simulink model "dtc_svpwm"  (Simulink 7.0)
settings: Solver=ode23tb  StartTime=0.0  StopTime=0.1  RelTol=1e-3
libraries: powerlib x4
settings Model: Creator=Administrator  LastModifiedBy=Administrator
settings SolverCC: ZeroCrossControl=DisableAll

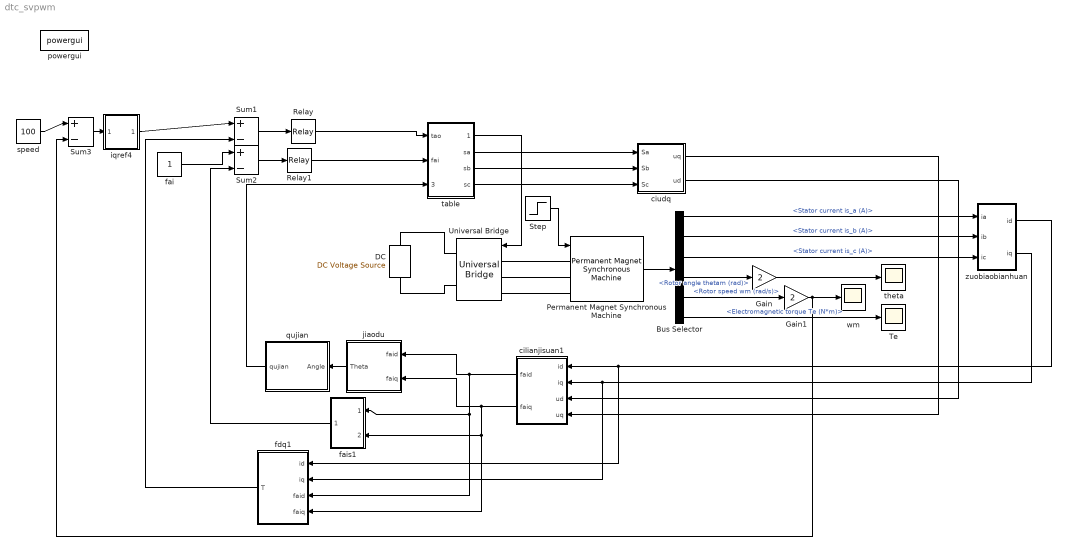
== system dtc_svpwm ==
  Bus Selector : BusSelector  OutputSignals=Stator current is_a (A),Stator current is_b (A),Stator current is_c (A),Rotor angle thetam (rad),Rotor speed wm (rad/s),Electromagnetic torque Te (N*m)
  "DC " : powerlib/Electrical Sources/DC Voltage Source  Orientation=up  DialogController=POWERSYS.PowerSysDialog  SystemSampleTime=-1  Amplitude=310  Measurements=None
  Gain : Gain  Gain=2  ParameterDataType=sfix(16)  ParameterScaling=2^0  OutDataType=sfix(16)  OutScaling=2^0
  Gain1 : Gain  Gain=2  ParameterDataType=sfix(16)  ParameterScaling=2^0  OutDataType=sfix(16)  OutScaling=2^0
  Permanent Magnet Synchronous Machine : powerlib/Machines/Permanent Magnet Synchronous Machine  DialogController=POWERSYS.PowerSysDialog  SystemSampleTime=-1  FluxDistribution=Sinusoidal  MechanicalLoad=Torque Tm  PresetModel=No  ShowDetailedParameters=on  Resistance=2.8750  Inductance=8.5e-3  dqInductances=[8.5e-3;8.5e-3]  Flux=0.3  Flat=120  Mechanical=[0.008 0 2]  PolePairs=2
  Relay : Relay  OnSwitchValue=0.001  OffSwitchValue=-0.001  OutDataType=sfix(16)  OutScaling=2^0
  Relay1 : Relay  OnSwitchValue=0.005  OffSwitchValue=-0.005  OutDataType=sfix(16)  OutScaling=2^0
  Step : Step  Time=0.04  Before=1  After=2  SampleTime=0
  Sum1 : Sum  Inputs=|+-  OutDataType=sfix(16)  OutScaling=2^0
  Sum2 : Sum  Inputs=|+-  OutDataType=sfix(16)  OutScaling=2^0
  Sum3 : Sum  Inputs=|+-  OutDataType=sfix(16)  OutScaling=2^0
  Te : Scope
      settings: YMin=-50  YMax=55
  Universal Bridge : powerlib/Power Electronics/Universal Bridge  Orientation=left  DialogController=POWERSYS.PowerSysDialog  SystemSampleTime=-1  Arms=3  SnubberResistance=1e5  SnubberCapacitance=inf  Device=IGBT / Diodes  Ron=1e-3  Lon=0  ForwardVoltages="[  0  0  ]"  ForwardVoltage=0  GTOparameters=[ 10e-6 , 20e-6 ]  IGBTparameters=[ 1e-6 , 2e-6 ]  Measurements=None  converterType=Rectifier
  cilianjisuan1 : Subsystem  Orientation=left
  ciudq : Subsystem
  fai : Constant  OutDataType=sfix(16)  OutScaling=2^0
  fais1 : Subsystem  Orientation=left
  fdq1 : Subsystem  Orientation=left
  iqref4 : Subsystem  mask(PI Controller){@1=0.02, @2=2, @3=[-3000, 3000]}
      mask prompts: @1 "Integral"; @2 "Proportional:"; @3 "Minimum and maximum outputs:"
      mask init:
      | I=@1;P=@2;sat=@3;min=sat(1);max=sat(2);
      mask Display: disp('PI')
  jiaodu : Subsystem  Orientation=left
  powergui : powerlib/powergui  SystemSampleTime=-1  SimulationMode=Continuous  SampleTime=50e-6  echomessages=off  RestoreLinks=warning  x0status=blocks  Frange=[0:2:500]  Ylog=off  Xlog=on  ShowGrid=off  save=off  variable=ZData  ZoomFFT=on  StartTime=0.0  cycles=1  DisplayStyle=1  fundamental=60  FreqAxis=off  MaxFrequency=1000  frequencyindice=0  frequencyindicesteady=1  RmsSteady=1  display=off  Ts=0  frequency=60  methode=off  HookPort=off  Interpol=off  SPID=off  FunctionMessages=off
  qujian : Subsystem  Orientation=left
  speed : Constant  Value=100  OutDataType=sfix(16)  OutScaling=2^0
  table : Subsystem
  theta : Scope
      settings: SaveName=ScopeData2
  wm : Scope
      settings: YMin=-100  YMax=110  SaveName=ScopeData3
  zuobiaobianhuan : Subsystem
      mask Type: bianhuan
  wires:
  table/1(Pulse) -> Universal Bridge/1
  Permanent Magnet Synchronous Machine/1 -> Bus Selector/1
  Bus Selector/4 -> Gain/1  "<Rotor angle thetam (rad)>"
  Gain/1 -> theta/1
  Bus Selector/6 -> Te/1  "<Electromagnetic torque Te (N*m)>"
  Gain1/1 -> wm/1, Sum3/2
  Step/1 -> Permanent Magnet Synchronous Machine/1
  Sum1/1 -> Relay/1
  Sum2/1 -> Relay1/1
  fais1/1(fais) -> Sum2/2
  fai/1 -> Sum2/1
  fdq1/1(T) -> Sum1/2
  jiaodu/1(Theta) -> qujian/1(Angle)
  cilianjisuan1/1(faid) -> jiaodu/1(faid), fdq1/3(faid), fais1/1(faid)
  cilianjisuan1/2(faiq) -> jiaodu/2(faiq), fdq1/4(faiq), fais1/2(faiq)
  table/3(sb) -> ciudq/2(Sb)
  speed/1 -> Sum3/1
  Bus Selector/5 -> Gain1/1  "<Rotor speed wm (rad/s)>"
  table/2(sa) -> ciudq/1(Sa)
  table/4(sc) -> ciudq/3(Sc)
  zuobiaobianhuan/1(id) -> fdq1/1(id), cilianjisuan1/1(id)
  zuobiaobianhuan/2(iq) -> fdq1/2(iq), cilianjisuan1/2(iq)
  Bus Selector/1 -> zuobiaobianhuan/1(ia)  "<Stator current is_a (A)>"
  Bus Selector/2 -> zuobiaobianhuan/2(ib)  "<Stator current is_b (A)>"
  Bus Selector/3 -> zuobiaobianhuan/3(ic)  "<Stator current is_c (A)>"
  Relay/1 -> table/1(tao)
  Relay1/1 -> table/2(fai)
  qujian/1(qujian) -> table/3(theta)
  Sum3/1 -> iqref4/1(In_1)
  iqref4/1(Out_1) -> Sum1/1
  ciudq/1(uq) -> cilianjisuan1/4(uq)
  ciudq/2(ud) -> cilianjisuan1/3(ud)
  connections:
  "DC "/RConn1 -- Universal Bridge/RConn1
  "DC "/LConn1 -- Universal Bridge/RConn2
  Universal Bridge/LConn1 -- Permanent Magnet Synchronous Machine/LConn1
  Universal Bridge/LConn2 -- Permanent Magnet Synchronous Machine/LConn2
  Universal Bridge/LConn3 -- Permanent Magnet Synchronous Machine/LConn3

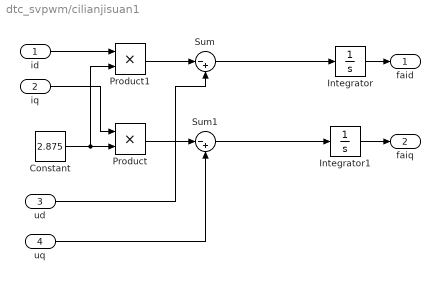
== system dtc_svpwm/cilianjisuan1 ==
  id : Inport  OutDataType=sfix(16)  OutScaling=2^0
  iq : Inport  Port=2  OutDataType=sfix(16)  OutScaling=2^0
  ud : Inport  Port=3  OutDataType=sfix(16)  OutScaling=2^0
  uq : Inport  Port=4  OutDataType=sfix(16)  OutScaling=2^0
  Constant : Constant  Value=2.875  OutDataType=sfix(16)  OutScaling=2^0
  Integrator : Integrator  InitialCondition=0.01
  Integrator1 : Integrator  InitialCondition=0.01
  Product : Product  OutDataType=sfix(16)  OutScaling=2^0  RndMeth=Zero
  Product1 : Product  OutDataType=sfix(16)  OutScaling=2^0  RndMeth=Zero
  Sum : Sum  Inputs=|-+  OutDataType=sfix(16)  OutScaling=2^0
  Sum1 : Sum  Inputs=|-+  OutDataType=sfix(16)  OutScaling=2^0
  faid : Outport  OutDataType=sfix(16)  OutScaling=2^0
  faiq : Outport  Port=2  OutDataType=sfix(16)  OutScaling=2^0
  wires:
  Integrator/1 -> faid/1
  Sum/1 -> Integrator/1
  Integrator1/1 -> faiq/1
  Sum1/1 -> Integrator1/1
  iq/1 -> Product/1
  Constant/1 -> Product/2, Product1/2
  id/1 -> Product1/1
  Product1/1 -> Sum/1
  Product/1 -> Sum1/1
  ud/1 -> Sum/2
  uq/1 -> Sum1/2

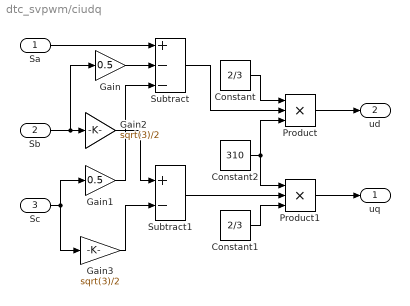
== system dtc_svpwm/ciudq ==
  Sa : Inport
  Sb : Inport  Port=2
  Sc : Inport  Port=3
  Constant : Constant  Value=2/3
  Constant1 : Constant  Value=2/3
  Constant2 : Constant  Value=310
  Gain : Gain  Gain=0.5
  Gain1 : Gain  Gain=0.5
  Gain2 : Gain  Gain=sqrt(3)/2
  Gain3 : Gain  Gain=sqrt(3)/2
  Product : Product  Inputs=3  RndMeth=Zero
  Product1 : Product  Inputs=3  RndMeth=Zero
  Subtract : Sum  Inputs=+--
  Subtract1 : Sum  Inputs=+-
  uq : Outport
  ud : Outport  Port=2
  wires:
  Sa/1 -> Subtract/1
  Gain/1 -> Subtract/2
  Sb/1 -> Gain2/1, Gain/1
  Sc/1 -> Gain3/1, Gain1/1
  Gain1/1 -> Subtract/3
  Gain2/1 -> Subtract1/1
  Gain3/1 -> Subtract1/2
  Subtract/1 -> Product/2
  Constant/1 -> Product/1
  Subtract1/1 -> Product1/2
  Constant1/1 -> Product1/3
  Constant2/1 -> Product1/1, Product/3
  Product/1 -> ud/1
  Product1/1 -> uq/1

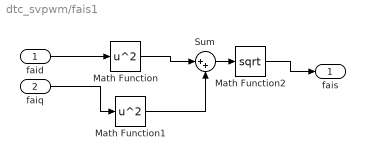
== system dtc_svpwm/fais1 ==
  faid : Inport  OutDataType=sfix(16)  OutScaling=2^0
  faiq : Inport  Port=2  OutDataType=sfix(16)  OutScaling=2^0
  Math Function : Math  Operator=square  OutDataType=sfix(16)  OutScaling=2^0  SaturateOnIntegerOverflow=on
  Math Function1 : Math  Operator=square  OutDataType=sfix(16)  OutScaling=2^0  SaturateOnIntegerOverflow=on
  Math Function2 : Math  Operator=sqrt  OutDataType=sfix(16)  OutScaling=2^0  SaturateOnIntegerOverflow=on
  Sum : Sum  Inputs=|++  OutDataType=sfix(16)  OutScaling=2^0
  fais : Outport  OutDataType=sfix(16)  OutScaling=2^0
  wires:
  faid/1 -> Math Function/1
  faiq/1 -> Math Function1/1
  Math Function2/1 -> fais/1
  Math Function/1 -> Sum/1
  Math Function1/1 -> Sum/2
  Sum/1 -> Math Function2/1

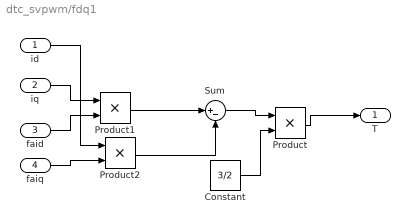
== system dtc_svpwm/fdq1 ==
  id : Inport  OutDataType=sfix(16)  OutScaling=2^0
  iq : Inport  Port=2  OutDataType=sfix(16)  OutScaling=2^0
  faid : Inport  Port=3  OutDataType=sfix(16)  OutScaling=2^0
  faiq : Inport  Port=4  OutDataType=sfix(16)  OutScaling=2^0
  Constant : Constant  Value=3/2  OutDataType=sfix(16)  OutScaling=2^0
  Product : Product  OutDataType=sfix(16)  OutScaling=2^0  RndMeth=Zero
  Product1 : Product  OutDataType=sfix(16)  OutScaling=2^0  RndMeth=Zero
  Product2 : Product  OutDataType=sfix(16)  OutScaling=2^0  RndMeth=Zero
  Sum : Sum  Inputs=|+-  OutDataType=sfix(16)  OutScaling=2^0
  T : Outport  OutDataType=sfix(16)  OutScaling=2^0
  wires:
  Sum/1 -> Product/1
  Constant/1 -> Product/2
  Product/1 -> T/1
  iq/1 -> Product1/1
  faid/1 -> Product1/2
  id/1 -> Product2/1
  faiq/1 -> Product2/2
  Product2/1 -> Sum/2
  Product1/1 -> Sum/1

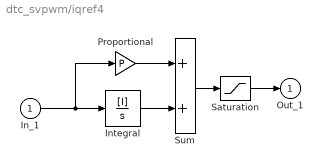
== system dtc_svpwm/iqref4 ==
  In_1 : Inport  OutDataType=sfix(16)  OutScaling=2^0
  Integral : TransferFcn  Numerator=[I]  Denominator=[1 0]
  Proportional : Gain  Gain=P  ParameterDataType=sfix(16)  ParameterScaling=2^0  OutDataType=sfix(16)  OutScaling=2^0  SaturateOnIntegerOverflow=on
  Saturation : Saturate  UpperLimit=max  LowerLimit=min
  Sum : Sum  OutDataType=sfix(16)  OutScaling=2^0  SaturateOnIntegerOverflow=on  InputSameDT=on
  Out_1 : Outport  OutDataType=sfix(16)  OutScaling=2^0  InitialOutput=0
  wires:
  Saturation/1 -> Out_1/1
  Sum/1 -> Saturation/1
  Proportional/1 -> Sum/1
  In_1/1 -> Proportional/1, Integral/1
  Integral/1 -> Sum/2

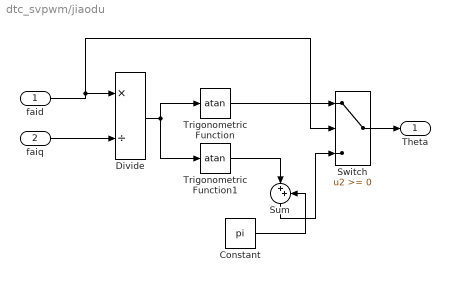
== system dtc_svpwm/jiaodu ==
  faid : Inport  OutDataType=sfix(16)  OutScaling=2^0
  faiq : Inport  Port=2  OutDataType=sfix(16)  OutScaling=2^0
  Constant : Constant  Value=pi  OutDataType=sfix(16)  OutScaling=2^0
  Divide : Product  Inputs=*/  OutDataType=sfix(16)  OutScaling=2^-10
  Sum : Sum  Orientation=down  Inputs=|++  OutDataType=sfix(16)  OutScaling=2^0
  Switch : Switch  OutDataType=sfix(16)  OutScaling=2^0
  Trigonometric Function : Trigonometry  Operator=atan
  Trigonometric Function1 : Trigonometry  Operator=atan
  Theta : Outport  OutDataType=sfix(16)  OutScaling=2^0
  wires:
  faid/1 -> Divide/1, Switch/2
  faiq/1 -> Divide/2
  Trigonometric Function/1 -> Switch/1
  Sum/1 -> Switch/3
  Constant/1 -> Sum/2
  Switch/1 -> Theta/1
  Divide/1 -> Trigonometric Function1/1, Trigonometric Function/1
  Trigonometric Function1/1 -> Sum/1

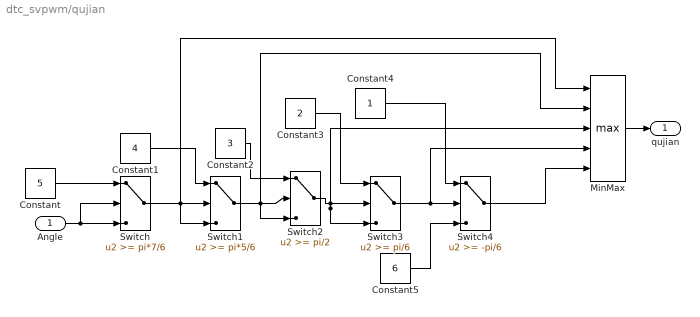
== system dtc_svpwm/qujian ==
  Angle : Inport  OutDataType=sfix(16)  OutScaling=2^0
  Constant : Constant  Value=5  OutDataType=sfix(16)  OutScaling=2^0
  Constant1 : Constant  Value=4  OutDataType=sfix(16)  OutScaling=2^0
  Constant2 : Constant  Value=3  OutDataType=sfix(16)  OutScaling=2^0
  Constant3 : Constant  Value=2  OutDataType=sfix(16)  OutScaling=2^0
  Constant4 : Constant  OutDataType=sfix(16)  OutScaling=2^0
  Constant5 : Constant  Value=6  OutDataType=sfix(16)  OutScaling=2^0
  MinMax : MinMax  Function=max  Inputs=5  OutDataType=sfix(16)  OutScaling=2^0
  Switch : Switch  Threshold=pi*7/6  OutDataType=sfix(16)  OutScaling=2^0
  Switch1 : Switch  Threshold=pi*5/6  OutDataType=sfix(16)  OutScaling=2^0
  Switch2 : Switch  Threshold=pi/2  OutDataType=sfix(16)  OutScaling=2^0
  Switch3 : Switch  Threshold=pi/6  OutDataType=sfix(16)  OutScaling=2^0
  Switch4 : Switch  Threshold=-pi/6  OutDataType=sfix(16)  OutScaling=2^0
  qujian : Outport  OutDataType=sfix(16)  OutScaling=2^0
  wires:
  Angle/1 -> Switch/3, Switch/2
  Constant/1 -> Switch/1
  Switch/1 -> Switch1/2, Switch1/3, MinMax/1
  Switch1/1 -> MinMax/2, Switch2/2, Switch2/3
  Constant1/1 -> Switch1/1
  Constant2/1 -> Switch2/1
  Constant3/1 -> Switch3/1
  Switch4/1 -> MinMax/5
  Constant4/1 -> Switch4/1
  MinMax/1 -> qujian/1
  Constant5/1 -> Switch4/3
  Switch2/1 -> Switch3/2, Switch3/3, MinMax/3
  Switch3/1 -> Switch4/2, MinMax/4

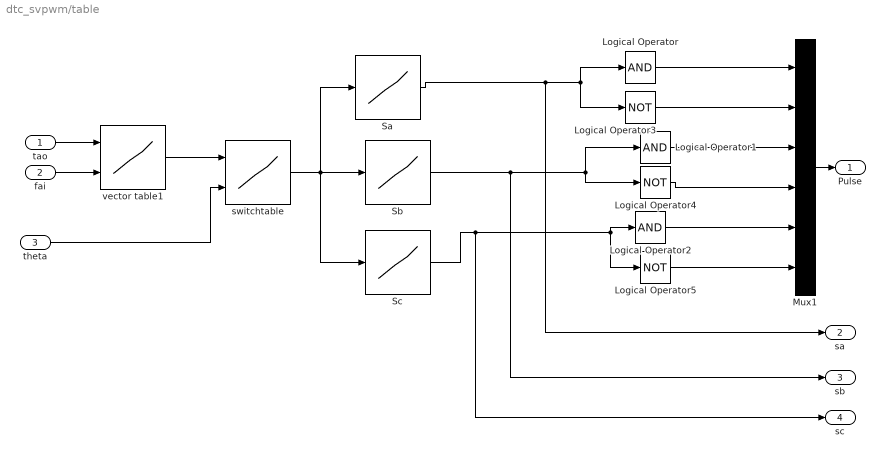
== system dtc_svpwm/table ==
  tao : Inport  OutDataType=sfix(16)  OutScaling=2^0
  fai : Inport  Port=2  OutDataType=sfix(16)  OutScaling=2^0
  theta : Inport  Port=3  OutDataType=sfix(16)  OutScaling=2^0
  Logical Operator : Logic  Inputs=1  AllPortsSameDT=off  OutDataTypeMode=boolean
  Logical Operator1 : Logic  Inputs=1  AllPortsSameDT=off  OutDataTypeMode=boolean
  Logical Operator2 : Logic  Inputs=1  AllPortsSameDT=off  OutDataTypeMode=boolean
  Logical Operator3 : Logic  Operator=NOT  Inputs=1  AllPortsSameDT=off  OutDataTypeMode=boolean
  Logical Operator4 : Logic  Operator=NOT  Inputs=1  AllPortsSameDT=off  OutDataTypeMode=boolean
  Logical Operator5 : Logic  Operator=NOT  Inputs=1  AllPortsSameDT=off  OutDataTypeMode=boolean
  Mux1 : Mux  Inputs=6
  Sa : Lookup_n-D  NumberOfTableDimensions=1  BreakpointsForDimension1=[1:6]  Table="[1 1  0 0 0 1]"
  Sb : Lookup_n-D  NumberOfTableDimensions=1  BreakpointsForDimension1=[1:6]  Table=[0 1 1 1 0 0]
  Sc : Lookup_n-D  NumberOfTableDimensions=1  BreakpointsForDimension1=[1,2,3,4,5,6]  Table=[0,0,0,1,1,1]
  switchtable : Lookup_n-D  BreakpointsForDimension1=[1:4]  BreakpointsForDimension2=[1:6]  Table=[2 3 4 5 6 1;6 1 2 3 4 5 ;3 4 5 6 1 2;5 6 1 2 3 4]
  vector table1 : Lookup_n-D  BreakpointsForDimension1=[0:1]  BreakpointsForDimension2=[0:1]  Table=[4 2;3 1]
  Pulse : Outport  OutDataType=sfix(16)  OutScaling=2^0
  sa : Outport  Port=2  OutDataType=sfix(16)  OutScaling=2^0
  sb : Outport  Port=3  OutDataType=sfix(16)  OutScaling=2^0
  sc : Outport  Port=4  OutDataType=sfix(16)  OutScaling=2^0
  wires:
  switchtable/1 -> Sa/1, Sc/1, Sb/1
  vector table1/1 -> switchtable/1
  tao/1 -> vector table1/1
  fai/1 -> vector table1/2
  theta/1 -> switchtable/2
  Sb/1 -> Logical Operator1/1, Logical Operator4/1, sb/1
  Sc/1 -> Logical Operator2/1, Logical Operator5/1, sc/1
  Sa/1 -> Logical Operator/1, Logical Operator3/1, sa/1
  Logical Operator3/1 -> Mux1/2
  Logical Operator4/1 -> Mux1/4
  Logical Operator5/1 -> Mux1/6
  Mux1/1 -> Pulse/1
  Logical Operator/1 -> Mux1/1
  Logical Operator1/1 -> Mux1/3
  Logical Operator2/1 -> Mux1/5

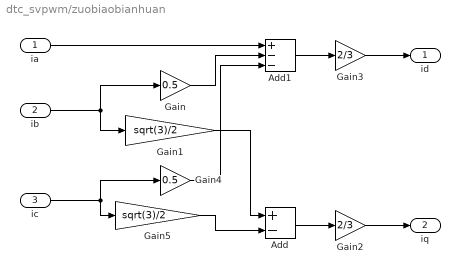
== system dtc_svpwm/zuobiaobianhuan ==
  ia : Inport
  ib : Inport  Port=2
  ic : Inport  Port=3
  Add : Sum  Inputs=+-
  Add1 : Sum  Inputs=+--
  Gain : Gain  Gain=0.5
  Gain1 : Gain  Gain=sqrt(3)/2
  Gain2 : Gain  Gain=2/3
  Gain3 : Gain  Gain=2/3
  Gain4 : Gain  Gain=0.5
  Gain5 : Gain  Gain=sqrt(3)/2
  id : Outport
  iq : Outport  Port=2
  wires:
  ic/1 -> Gain5/1, Gain4/1
  ib/1 -> Gain1/1, Gain/1
  Gain1/1 -> Add/1
  Gain4/1 -> Add1/3
  Gain/1 -> Add1/2
  ia/1 -> Add1/1
  Gain5/1 -> Add/2
  Gain3/1 -> id/1
  Gain2/1 -> iq/1
  Add/1 -> Gain2/1
  Add1/1 -> Gain3/1
